simulink model "SimForcesGP2017a"  (R2020b)
settings: Solver=ode4  StartTime=0.0  StopTime=10  FixedStep=0.001  MaxStep=0.001  RelTol=1e-7
values from neighbouring files (symbols this model uses):
  B11_r_B11C = [0.23805608; 0.13201777; 0]    [InitializeSimulationGP.m]
  B11_r_B11Tc1 = [L11; 0; 0]    [InitializeSimulationGP.m]
  B11_Rot_Tc1 = eye(3)    [InitializeSimulationGP.m]
  B11cI = [0.28426000 -0.06487287 0;         -0.06487287  0.54237481 0;                   0  0          0.67891020]    [InitializeSimulationGP.m]
  B12_r_B12C = [0.60504569; 0.27199376; 0.00002484]    [InitializeSimulationGP.m]
  B12_r_B12Tc2 = [L21;0;0]    [InitializeSimulationGP.m]
  B12_Rot_Tc2 = eye(3)    [InitializeSimulationGP.m]
  B12cI = [1.18803886 -2.36786418 0.00280315;          -2.36786418 6.31493281 0.00022322;           0.00280315 0.00022322 7.40915161]    [InitializeSimulationGP.m]
  B31_r_B31C = [0.35781210 0 0]    [InitializeSimulationGP.m]
  B31_Rot_B41 = eye(3)    [InitializeSimulationGP.m]
  B31cI = diag([0.03150902 0.90735702 0.90763033])    [InitializeSimulationGP.m]
  B32_r_B32C = [0.35781210 0 0]    [InitializeSimulationGP.m]
  B32_Rot_B42 = eye(3)    [InitializeSimulationGP.m]
  B32cI = diag([0.03150902 0.90735702 0.90763033])    [InitializeSimulationGP.m]
  B41_r_B41C = [0.55785997 0 0]    [InitializeSimulationGP.m]
  B41_r_B41Tc1 = [lc1;0;0]    [InitializeSimulationGP.m]
  B41cI = diag([0.00370720 0.55759812 0.55785997])    [InitializeSimulationGP.m]
  B42_r_B42C = [0.55785997 0 0]    [InitializeSimulationGP.m]
  B42_r_B42Tc2 = [lc2; 0; 0]    [InitializeSimulationGP.m]
  B42cI = diag([0.00370720 0.55759812 0.55785997])    [InitializeSimulationGP.m]
  B52_r_B52C = [0 0 0.56802906]    [InitializeSimulationGP.m]
  B52_r_B52P32 = [lc3; 0; 0]    [InitializeSimulationGP.m]
  B52_Rot_P32 = eye(3)    [InitializeSimulationGP.m]
  B52cI = diag([0.91789884, 0.91790043, 0.00091463])    [InitializeSimulationGP.m]
  Bc1_r_Bc1B11 = [L1; 0; 0]    [InitializeSimulationGP.m]
  Bc1_r_Bc1B31 = [0;0;0]    [InitializeSimulationGP.m]
  Bc1_r_Bc1C = [0.14178771; 0.16555780; 0]    [InitializeSimulationGP.m]
  Bc1_V = [0;0;0;0;0;0]    [InitializeSimulationGP.m]
  Bc1cI = [+5.892211080 +5.476111360 -0.000019630;          +5.476111360 +28.66965601 -0.000024550;          -0.000019630 -0.000024550 +29.78955950]    [InitializeSimulationGP.m]
  Bc2_r_Bc2B12 = [L2;0;0]    [InitializeSimulationGP.m]
  Bc2_r_Bc2B32 = [0;0;0]    [InitializeSimulationGP.m]
  Bc2_r_Bc2C = [0.54319901; 0.10543875; 0]    [InitializeSimulationGP.m]
  Bc2cI = [0.48071390 0.52924041 0;          0.52924041 5.80912352 0;              0      0          5.97255351]    [InitializeSimulationGP.m]
  beta1 = atan2d(374.261,935)*pi/180    [InitializeSimulationGP.m]
  beta2 = atan2d(45.757,373.313)*pi/180    [InitializeSimulationGP.m]
  beta3 = atan2d(139.50,1132.19)*pi/180    [InitializeSimulationGP.m]
  beta4 = atan2d(88.061,296.198)*pi/180    [InitializeSimulationGP.m]
  D22F = [0;0;0;0;0;0]    [InitializeSimulationGP.m]
  L1 = 1.0071227324212    (= 1.00712273242)    [InitializeSimulationGP.m]
  L11 = 0.37610632101293    (= 0.376106321013)    [InitializeSimulationGP.m]
  L2 = 1.132185817991    (= 1.13218581799)    [InitializeSimulationGP.m]
  L21 = 0.30901132665325    (= 0.309011326653)    [InitializeSimulationGP.m]
  lc1 = 0.745    [InitializeSimulationGP.m]
  lc2 = 0.745    [InitializeSimulationGP.m]
  mB11 = 25.52660174    [InitializeSimulationGP.m]
  mB12 = 33.92850233    [InitializeSimulationGP.m]
  mB31 = 17.36281648    [InitializeSimulationGP.m]
  mB32 = 17.36281648    [InitializeSimulationGP.m]
  mB41 = 10.34519231    [InitializeSimulationGP.m]
  mB42 = 10.34519231    [InitializeSimulationGP.m]
  mB52 = 6.73059863    [InitializeSimulationGP.m]
  mBc1 = 307.29601379    [InitializeSimulationGP.m]
  mBc2 = 54.58702836    [InitializeSimulationGP.m]
  mP22 = 9.26136143    [InitializeSimulationGP.m]
  mP32 = 570.18877059    [InitializeSimulationGP.m]
  P22_r_P22C = [0.62192523 0 0]    [InitializeSimulationGP.m]
  P22_Rot_B52 = eye(3)    [InitializeSimulationGP.m]
  P22cI = diag([0.00662754, 1.48387017, 1.48398069])    [InitializeSimulationGP.m]
  P32_r_P32C = [0.25466704; -0.13034397; -0.01302248]    [InitializeSimulationGP.m]
  P32_r_P32D22 = [0.40499744871392; -0.13130517281345; -0.013385243295654]    [InitializeSimulationGP.m]
  P32_Rot_D22 = [1 0 0;              0 0.9707729441837 0.23999977258512;              0 -0.23999977258512 0.9707729441837]    [InitializeSimulationGP.m]
  P32cI = [46.81220713 0.38607676 -0.00453819;          0.38607676 71.92201786 -1.14320993;          -0.00453819 -1.14320993 67.38128576]    [InitializeSimulationGP.m]
  Tc1_r_Tc1Bc2 = [0.098495302558553; 0.01838181329939; 0]    [InitializeSimulationGP.m]
  Tc1_Rot_Bc2 = [cos(alpha2) -sin(alpha2) 0;                sin(alpha2)  cos(alpha2) 0;                0            0           1]    [InitializeSimulationGP.m]
  Tc2_r_Tc2P22 = [-0.048858374920227;0.36587359346146;0.035276938723102]    [InitializeSimulationGP.m]
  Tc2_Rot_P22 = [0.95853460763586 -0.27664713597974  0.0683942111482;                0.28497614981675  0.93051946315663 -0.23004808784757;                0                 0.23999977258511  0.9707729441837]    [InitializeSimulationGP.m]
  Th1A = 5*pi/180    (= 0.0872664625997)    [InitializeSimulationGP.m]
  Th1B = 20*pi/180    (= 0.349065850399)    [InitializeSimulationGP.m]
  Th1f = 1    [InitializeSimulationGP.m]
  Th2A = 15*pi/180    (= 0.261799387799)    [InitializeSimulationGP.m]
  Th2B = -50*pi/180    (= -0.872664625997)    [InitializeSimulationGP.m]
  Th2f = 2    [InitializeSimulationGP.m]
  W_r_WBc1 = [0.185;-0.085;0]    [InitializeSimulationGP.m]
  W_Rot_Bc1 = [cos(alpha1) -sin(alpha1) 0;              sin(alpha1)  cos(alpha1) 0;              0            0           1]    [InitializeSimulationGP.m]
  Wg = [0; 9.8066; 0]    [InitializeSimulationGP.m]
  x10 = 0.83    [InitializeSimulationGP.m]
  x20 = 0.83    [InitializeSimulationGP.m]
  xf = [1;0;0;0;0;0]    [InitializeSimulationGP.m]
  xt2A = 0.1    [InitializeSimulationGP.m]
  xt2B = 0.5    [InitializeSimulationGP.m]
  xt2f = 1    [InitializeSimulationGP.m]
  ztau = [0;0;0;0;0;1]    [InitializeSimulationGP.m]
undefined symbols (not defined in the file or in its folder): B11_V, B11_V_SS, B11Ftot, B12_U_Tc2, B12_V, B12_V_SS, B12Ftot, B31_r_B31B41, B31_V, B31_V_SS, B31FTot, B32_r_B32B42, B32_U_B42, B32_V, B32_V_SS, B32FTot, B41_V, B41_V_SS, B41FTot, B42_Rot_Tc2, B42_U_Tc2, B42_V, B42_V_SS, B42FTot, B52_U_P32, B52_V, B52_V_SS, B52Ftot, Bc1_V_SS, Bc1Tot, Bc2_Rot_B12, Bc2_Rot_B32, Bc2_U_B12, Bc2_U_B32, Bc2_V, Bc2_V_SS, Bc2Tot, D22_V, D22_V_SS, dq1, dq11, dq12, dq2, dq21, dq22, dx1, dx2, FTot_S1, FTot_S2P, FTot_S2R, P22_r_P22B52, P22_U_B52, P22_V, P22_V_SS, P22FTot, P32_U_D22, P32_V, P32_V_SS, P32FTot, q1 ... (+28)
libraries: nesl_utility x94, sm_lib x45
(part 1 of 5)
settings Model: Creator=liikaneh  LastModifiedBy=Goran
settings OptimizationCC: DefaultParameterBehavior=Inlined  UseFloatMulNetSlope=on  InlineInvariantSignals=on  EfficientFloat2IntCast=on
settings DebuggingCC: ReadBeforeWriteMsg=DisableAll  WriteAfterWriteMsg=DisableAll  WriteAfterReadMsg=DisableAll  MultiTaskDSMMsg=none  ArithmeticOperatorsInVariantConditions=warning
settings ModelReferenceCC: UpdateModelReferenceTargets=IfOutOfDate
settings SFSimCC: SFSimEcho=off  SimUseLocalCustomCode=off  CustomCodeUndefinedFunction=UseInterfaceOnly
settings RTWCC: RTWUseLocalCustomCode=off  BuildConfiguration=Faster Runs
settings CodeAppCC: StateflowObjectComments=on
settings GRTTargetCC: MatFileLogging=off  SupportNonFinite=off
settings DiagnosticsConfigSet: SimMechanicsRigidlyBoundBlock=none

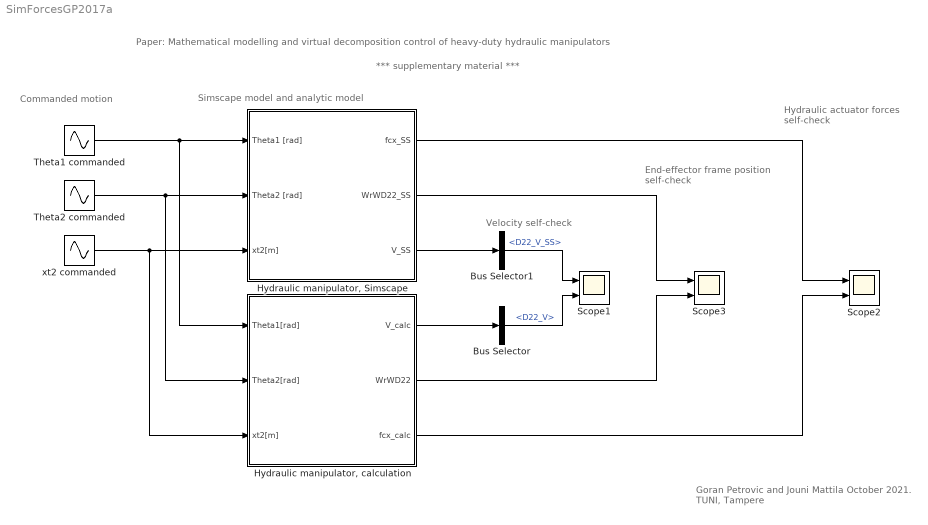
== system SimForcesGP2017a ==
  note: *** supplementary material ***
  note: Paper: Mathematical modelling and virtual decomposition control of heavy-duty hydraulic manipulators
  note: Commanded motion
  note: Simscape model and analytic model
  note: Hydraulic actuator
      | forces self-check
  note: End-effector frame
      | position self-check
  note: Velocity self-check
  note: Goran Petrovic and Jouni Mattila
      | October 2021.
      | TUNI, Tampere
  Bus Selector : BusSelector  OutputSignals=Vels_S2P.D22_V
  Bus Selector1 : BusSelector  OutputSignals=D22_V_SS
  "Hydraulic manipulator, Simscape" : Subsystem
  "Hydraulic manipulator, calculation" : Subsystem
  Scope1 : Scope  NumInputPorts=2
  Scope2 : Scope  NumInputPorts=2
  Scope3 : Scope  NumInputPorts=2
  Theta1 commanded : Sin  Amplitude=Th1A  Bias=Th1B  Frequency=Th1f  SampleTime=0
  Theta2 commanded : Sin  Amplitude=Th2A  Bias=Th2B  Frequency=Th2f  SampleTime=0
  xt2 commanded : Sin  Amplitude=xt2A  Bias=xt2B  Frequency=xt2f  SampleTime=0
  wires:
  xt2 commanded/1 -> "Hydraulic manipulator, calculation"/3(xt2[m]), "Hydraulic manipulator, Simscape"/3(xt2[m])
  Theta1 commanded/1 -> "Hydraulic manipulator, calculation"/1(Theta1[rad]), "Hydraulic manipulator, Simscape"/1(Theta1 [rad])
  Theta2 commanded/1 -> "Hydraulic manipulator, calculation"/2(Theta2[rad]), "Hydraulic manipulator, Simscape"/2(Theta2 [rad])
  "Hydraulic manipulator, calculation"/1(V_calc) -> Bus Selector/1
  "Hydraulic manipulator, Simscape"/3(V_SS) -> Bus Selector1/1
  Bus Selector/1 -> Scope1/2  "<D22_V>"
  Bus Selector1/1 -> Scope1/1  "<D22_V_SS>"
  "Hydraulic manipulator, Simscape"/1(fcx_SS) -> Scope2/1
  "Hydraulic manipulator, calculation"/3(fcx_calc) -> Scope2/2
  "Hydraulic manipulator, Simscape"/2(WrWD22_SS) -> Scope3/1
  "Hydraulic manipulator, calculation"/2(WrWD22) -> Scope3/2

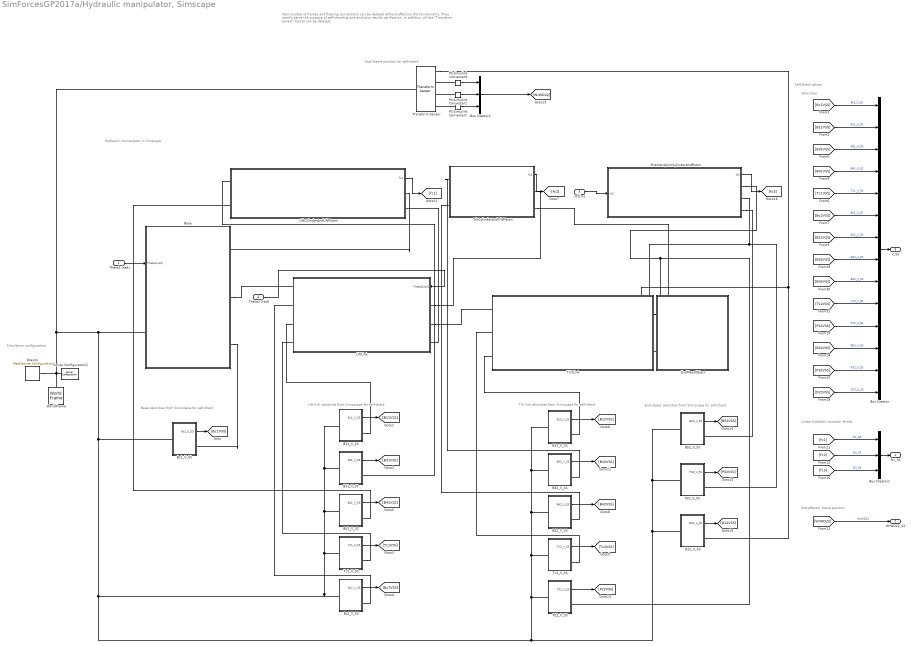
== system SimForcesGP2017a/Hydraulic manipulator, Simscape ==
  note: Vast number of frames and floating connections can be deleted without affecting the functionality.
      | They mainly serve the purpose of self-checking and analytics results verification.
      | In addition, all the "Transform sensor" blocks can be deleted.
  note: Hydraulic manipulator in Simscape
  note: Simulation configuration
  note: End object velocities from Simcscape for self-check
  note: Tilt link velocities from Simcscape for self-check
  note: Base velocities from Simcscape for self-check
  note: Lift link velocities from Simcscape for self-check
  note: Self-check values
  note: Velocities
  note: Linear hydraulic actuator forces
  note: End-effector frame position
  note: Goal frame position for self-check
  Theta1 [rad] : Inport
  Theta2 [rad] : Inport  Port=2
  xt2[m] : Inport  Port=3
  B11_V_SS : Subsystem
  B12_V_SS : Subsystem
  B31_V_SS : Subsystem
  B32_V_SS : Subsystem
  B41_V_SS : Subsystem
  B42_V_SS : Subsystem
  B52_V_SS : Subsystem
  Base : Subsystem
  Bc1_V_SS : Subsystem
  Bc2_V_SS : Subsystem
  Bus Creator : BusCreator  Inputs=Bc1_V_SS,B11_V_SS,B31_V_SS,B41_V_SS,Tc1_V_SS,Bc2_V_SS,B12_V_SS,B32_V_SS,B42_V_SS,Tc2_V_SS,P22_V_SS,B52_V_SS,P32_V_SS,D22_V_SS
  Bus Creator1 : BusCreator  Inputs=3
  Bus Creator2 : BusCreator  Inputs=3
  D22_V_SS : Subsystem
  EndMassObject : Subsystem
  Gravity : sm_lib/Utilities/Mechanism Configuration  UniformGravity=Constant  GravityVector=-Wg  GravityVectorUnits=m/s^2  GravityUnits=m/s^2  LinearizationDelta=0.001  JointModeTransitionNonlinearIterations=2
  LiftCylinderAndLiftPiston : Subsystem
  LiftLink : Subsystem
  P22_V_SS : Subsystem
  P32_V_SS : Subsystem
  PS-Simulink Converter1 : nesl_utility/PS-Simulink Converter  PhysicalDomain=network_engine_domain  SubClassName=ps_output  LeftPortType=input  RightPortType=output  PseudoPeriodic=off  Frequencies=[]  Unit=inherit  AffineConversion=off
  PS-Simulink Converter2 : nesl_utility/PS-Simulink Converter  PhysicalDomain=network_engine_domain  SubClassName=ps_output  LeftPortType=input  RightPortType=output  PseudoPeriodic=off  Frequencies=[]  Unit=inherit  AffineConversion=off
  PS-Simulink Converter8 : nesl_utility/PS-Simulink Converter  PhysicalDomain=network_engine_domain  SubClassName=ps_output  LeftPortType=input  RightPortType=output  PseudoPeriodic=off  Frequencies=[]  Unit=inherit  AffineConversion=off
  PrismaticJointCylinderAndPiston : Subsystem
  Solver Configuration1 : nesl_utility/Solver Configuration  PhysicalDomain=network_engine_domain  SubClassName=solver  LeftPortType=input  RightPortType=generic  Tones=[]  Harmonics=[]  SimulateNoise=off  Profile=off  UseLocalSampling=off  EnableSwitchedLinearOptims=on  FrequencyDomain=off  UseCCode=off  RelTol=0.001  AbsTol=1e-06  MinStep=1e-09  ToWorkspace=off  RevertToSquareIcSolve=off  NumHomotopyIterations=100  PhasorMode=off  PhasorModeNumHarmonics=1  DoDC=on  ResidualTolerance=1e-9  UseLocalSolver=off  LocalSolverChoice=NE_TRAPEZOIDAL_ADVANCER  LocalSolverSampleTime=0.002  DoFixedCost=off  MaxNonlinIter=3  MaxModeIter=2  ComputeImpulses=off  ImpulseIterations=2  LinearAlgebra=Sparse  EquationFormulation=NE_TIME_EF  DelaysMemoryBudget=1024  AutomaticFiltering=on  FilteringTimeConstant=0.001  PartitionStorageMethod=AS_NEEDED  PartitionMemoryBudget=1024  PartitionMethod=FAST
  Tc1_V_SS : Subsystem
  Tc2_V_SS : Subsystem
  TilitLink : Subsystem
  TiltCylinderAndTiltPiston : Subsystem
  Transform Sensor : sm_lib/Frames and Transforms/Transform Sensor  MeasurementFrame=NonRotatingBase  SenseAngle=off  SenseAxis=off  SenseAngle1=off  SenseAngle2=off  SenseAngle3=off  SenseQ=off  SenseR=off  SenseOmegaX=off  SenseOmegaY=off  SenseOmegaZ=off  SenseOmega1=off  SenseOmega2=off  SenseOmega3=off  SenseQDot=off  SenseRDot=off  SenseAlphaX=off  SenseAlphaY=off  SenseAlphaZ=off  SenseAlpha1=off  SenseAlpha2=off  SenseAlpha3=off  SenseQDDot=off  SenseRDDot=off  SenseX=on  SenseY=on  SenseZ=on  SenseRad=off  SenseAzim=off  SenseDist=off  SenseInc=off  SenseXDot=off  SenseYDot=off  SenseZDot=off  SenseRadDot=off  SenseAzimDot=off  SenseDistDot=off  SenseIncDot=off  SenseXDDot=off  SenseYDDot=off  SenseZDDot=off  SenseRadDDot=off  SenseAzimDDot=off  SenseDistDDot=off  SenseIncDDot=off
  WorldFrame : sm_lib/Frames and Transforms/World Frame
  fcx_SS : Outport
  WrWD22_SS : Outport  Port=2
  V_SS : Outport  Port=3
  wires:
  LiftCylinderAndLiftPiston/1(fc1) -> [fc1]
  TiltCylinderAndTiltPiston/1(fc2) -> [fc2]
  xt2[m]/1 -> PrismaticJointCylinderAndPiston/1(xt2)
  PrismaticJointCylinderAndPiston/1(fc3) -> [fc3]
  Theta1 [rad]/1 -> Base/1(Theta1[rad])
  Theta2 [rad]/1 -> LiftLink/1(Theta2[rad])
  B11_V_SS/1(B11_V_SS) -> [B11VSS]
  B41_V_SS/1(B41_V_SS) -> [B41VSS]
  B52_V_SS/1(B52_V_SS) -> [B52VSS]
  Bc1_V_SS/1(Bc1_V_SS) -> [Bc1VSS]
  B12_V_SS/1(B12_V_SS) -> [B12VSS]
  P32_V_SS/1(P32_V_SS) -> [P32VSS]
  P22_V_SS/1(P22_V_SS) -> [P22VSS]
  Tc2_V_SS/1(Tc2_V_SS) -> [Tc2VSS]
  B31_V_SS/1(B31_V_SS) -> [B31VSS]
  B42_V_SS/1(B42_V_SS) -> [B42VSS]
  D22_V_SS/1(D22_V_SS) -> [D22VSS]
  Bc2_V_SS/1(Bc2_V_SS) -> [Bc2VSS]
  Tc1_V_SS/1(Tc1_V_SS) -> [Tc1VSS]
  B32_V_SS/1(B32_V_SS) -> [B32VSS]
  [B12VSS] -> Bus Creator/7  "B12_V_SS"
  [B42VSS] -> Bus Creator/9  "B42_V_SS"
  [Tc2VSS] -> Bus Creator/10  "Tc2_V_SS"
  [fc1] -> Bus Creator1/1  "fc1_SS"
  Bus Creator/1 -> V_SS/1
  [P32VSS] -> Bus Creator/13  "P32_V_SS"
  [B32VSS] -> Bus Creator/8  "B32_V_SS"
  [fc2] -> Bus Creator1/2  "fc2_SS"
  [fc3] -> Bus Creator1/3  "fc3_SS"
  [WrWD22] -> WrWD22_SS/1  "WrWD22"
  Bus Creator1/1 -> fcx_SS/1
  [B52VSS] -> Bus Creator/12  "B52_V_SS"
  [P22VSS] -> Bus Creator/11  "P22_V_SS"
  [D22VSS] -> Bus Creator/14  "D22_V_SS"
  [Bc1VSS] -> Bus Creator/1  "Bc1_V_SS"
  [B11VSS] -> Bus Creator/2  "B11_V_SS"
  [Tc1VSS] -> Bus Creator/5  "Tc1_V_SS"
  [B41VSS] -> Bus Creator/4  "B41_V_SS"
  [B31VSS] -> Bus Creator/3  "B31_V_SS"
  [Bc2VSS] -> Bus Creator/6  "Bc2_V_SS"
  PS-Simulink Converter2/1 -> Bus Creator2/3
  PS-Simulink Converter8/1 -> Bus Creator2/1
  PS-Simulink Converter1/1 -> Bus Creator2/2
  Bus Creator2/1 -> [WrWD22]
  connections:
  P32_V_SS/LConn1 -- B52_V_SS/LConn1 -- Gravity/RConn1 -- WorldFrame/RConn1 -- Solver Configuration1/RConn1 -- Transform Sensor/LConn1 -- Base/LConn1 -- Bc1_V_SS/LConn1 -- B41_V_SS/LConn1 -- B31_V_SS/LConn1 -- B11_V_SS/LConn1 -- Tc1_V_SS/LConn1 -- Bc2_V_SS/LConn1 -- B32_V_SS/LConn1 -- B12_V_SS/LConn1 -- B42_V_SS/LConn1 -- Tc2_V_SS/LConn1 -- P22_V_SS/LConn1 -- D22_V_SS/LConn1
  LiftLink/LConn1 -- TiltCylinderAndTiltPiston/RConn1
  LiftLink/LConn2 -- TilitLink/RConn1
  TiltCylinderAndTiltPiston/RConn2 -- TilitLink/LConn2
  LiftCylinderAndLiftPiston/RConn2 -- LiftLink/LConn3
  Base/RConn2 -- LiftLink/RConn1
  LiftCylinderAndLiftPiston/RConn1 -- Base/RConn1
  Tc1_V_SS/RConn1 -- LiftLink/RConn4
  PrismaticJointCylinderAndPiston/RConn2 -- EndMassObject/LConn1 -- P32_V_SS/RConn1
  EndMassObject/LConn2 -- Transform Sensor/RConn1 -- D22_V_SS/RConn1
  LiftCylinderAndLiftPiston/LConn2 -- B41_V_SS/RConn1
  B11_V_SS/RConn1 -- LiftLink/RConn3
  TiltCylinderAndTiltPiston/LConn2 -- B42_V_SS/RConn1
  TiltCylinderAndTiltPiston/LConn1 -- B32_V_SS/RConn1
  PrismaticJointCylinderAndPiston/RConn1 -- P22_V_SS/RConn1 -- TilitLink/LConn1
  LiftCylinderAndLiftPiston/LConn1 -- B31_V_SS/RConn1
  TilitLink/RConn3 -- B12_V_SS/RConn1
  PrismaticJointCylinderAndPiston/RConn3 -- B52_V_SS/RConn1
  LiftLink/RConn2 -- Bc2_V_SS/RConn1
  Tc2_V_SS/RConn1 -- TilitLink/RConn2
  Base/RConn3 -- Bc1_V_SS/RConn1
  PS-Simulink Converter1/LConn1 -- Transform Sensor/RConn3
  PS-Simulink Converter8/LConn1 -- Transform Sensor/RConn2
  PS-Simulink Converter2/LConn1 -- Transform Sensor/RConn4

== system SimForcesGP2017a/Hydraulic manipulator, calculation ==
  note: Pass to outputs...
  note: Get inputs...
  note: Process data...
  Theta1[rad] : Inport
  Theta2[rad] : Inport  Port=2
  xt2[m] : Inport  Port=3
  AnalyticEnd-EffectorFramePosition : Subsystem
  AnalyticForces : Subsystem
  AnalyticTotalForces : Subsystem
  AnalyticVelocities : Subsystem
  AngleRelations : Subsystem
  Constant1 : Constant  Value=Bc1_V
  D22F : Constant  Value=D22F
  V_calc : Outport
  WrWD22 : Outport  Port=2
  fcx_calc : Outport  Port=3
  wires:
  AnalyticTotalForces/1(FTot_Sx) -> [FTot_Sx]
  AnalyticVelocities/1(GeomProp_Sx) -> [GeomSx]
  AnalyticVelocities/4(UMat_Sx) -> [UMatsSx]
  [UMatsSx] -> AnalyticForces/2(UMatSx)
  [VelsSx] -> AnalyticTotalForces/1(Vels_Sx)
  [GeomSx] -> AnalyticForces/3(GeomCCx)
  AnalyticVelocities/3(WRotX_Sx) -> [WRotXSx]
  [WRotXSx] -> AnalyticTotalForces/2(WRotX_Sx)
  [FTot_Sx] -> AnalyticForces/1(Ftot_Sx)
  AnalyticVelocities/5(Vels_Sx) -> [VelsSx]
  Theta1[rad]/1 -> [Theta1]  "Theta1"
  Theta2[rad]/1 -> [Theta2]  "Theta2"
  [Theta1] -> AngleRelations/1(Theta1[rad])  "Theta1"
  [Theta2] -> AngleRelations/2(Theta2[rad])  "Theta2"
  AngleRelations/1(q1[rad]) -> [q1]  "q1"
  AngleRelations/2(q2[rad]) -> [q2]  "q2"
  [q2] -> AnalyticVelocities/2(q2[rad])  "q2"
  [q1] -> AnalyticVelocities/1(q1[rad])  "q1"
  AnalyticForces/1(fc) -> [fc]
  [fc] -> fcx_calc/1
  [VelsSx] -> V_calc/1
  [D22F] -> AnalyticForces/4(GF)
  [WRotXSx] -> AnalyticEnd-EffectorFramePosition/2(WRotX_Sx)
  AnalyticVelocities/2(PosVecs_Sx) -> [PosVecsSx]
  [PosVecsSx] -> AnalyticEnd-EffectorFramePosition/1(PosVecs_Sx)
  AnalyticEnd-EffectorFramePosition/1(WrWD22) -> [WrWD22]
  [WrWD22] -> WrWD22/1
  D22F/1 -> [D22F]  "D22F"
  xt2[m]/1 -> [xt2]  "xt2"
  [xt2] -> AnalyticVelocities/3(xt2[m])  "x3"
  Constant1/1 -> [Bc1V]  "Bc1_V"
  [Bc1V] -> AnalyticVelocities/4(Bc1V)

== system SimForcesGP2017a/Hydraulic manipulator, Simscape/B11_V_SS ==
  Mux3 : Mux  Inputs=6
  PS-Simulink Converter{1..3,7..9} (6 alike) : nesl_utility/PS-Simulink Converter  PhysicalDomain=network_engine_domain  SubClassName=ps_output  LeftPortType=input  RightPortType=output  PseudoPeriodic=off  Frequencies=[]  Unit=inherit  AffineConversion=off
  Selector : Selector  InputPortWidth=6  IndexOptions=Index vector (dialog)  Indices=[4 5 6 1 2 3]  OutputSizes=1
  Transform Sensor3 : sm_lib/Frames and Transforms/Transform Sensor  MeasurementFrame=NonRotatingFollower  SenseAngle=off  SenseAxis=off  SenseAngle1=off  SenseAngle2=off  SenseAngle3=off  SenseQ=off  SenseR=off  SenseOmegaX=on  SenseOmegaY=on  SenseOmegaZ=on  SenseOmega1=off  SenseOmega2=off  SenseOmega3=off  SenseQDot=off  SenseRDot=off  SenseAlphaX=off  SenseAlphaY=off  SenseAlphaZ=off  SenseAlpha1=off  SenseAlpha2=off  SenseAlpha3=off  SenseQDDot=off  SenseRDDot=off  SenseX=off  SenseY=off  SenseZ=off  SenseRad=off  SenseAzim=off  SenseDist=off  SenseInc=off  SenseXDot=on  SenseYDot=on  SenseZDot=on  SenseRadDot=off  SenseAzimDot=off  SenseDistDot=off  SenseIncDot=off  SenseXDDot=off  SenseYDDot=off  SenseZDDot=off  SenseRadDDot=off  SenseAzimDDot=off  SenseDistDDot=off  SenseIncDDot=off
  Lift_B11 : PMIOPort  Side=Right
  W : PMIOPort  Port=2  Side=Left
  B11_V_SS : Outport
  wires:
  Mux3/1 -> Selector/1
  PS-Simulink Converter7/1 -> Mux3/2
  PS-Simulink Converter3/1 -> Mux3/6
  PS-Simulink Converter2/1 -> Mux3/5
  PS-Simulink Converter9/1 -> Mux3/1
  PS-Simulink Converter8/1 -> Mux3/3
  PS-Simulink Converter1/1 -> Mux3/4
  Selector/1 -> B11_V_SS/1
  connections:
  Transform Sensor3/RConn5 -- PS-Simulink Converter1/LConn1
  PS-Simulink Converter3/LConn1 -- Transform Sensor3/RConn7
  Transform Sensor3/LConn1 -- W/RConn1
  Transform Sensor3/RConn4 -- PS-Simulink Converter8/LConn1
  PS-Simulink Converter7/LConn1 -- Transform Sensor3/RConn3
  PS-Simulink Converter9/LConn1 -- Transform Sensor3/RConn2
  Transform Sensor3/RConn6 -- PS-Simulink Converter2/LConn1
  Transform Sensor3/RConn1 -- Lift_B11/RConn1

== system SimForcesGP2017a/Hydraulic manipulator, Simscape/B12_V_SS ==
  Mux3 : Mux  Inputs=6
  PS-Simulink Converter{1..3,7..9} (6 alike) : nesl_utility/PS-Simulink Converter  PhysicalDomain=network_engine_domain  SubClassName=ps_output  LeftPortType=input  RightPortType=output  PseudoPeriodic=off  Frequencies=[]  Unit=inherit  AffineConversion=off
  Selector1 : Selector  InputPortWidth=6  IndexOptions=Index vector (dialog)  Indices=[4 5 6 1 2 3]  OutputSizes=1
  Transform Sensor1 : sm_lib/Frames and Transforms/Transform Sensor  MeasurementFrame=NonRotatingFollower  SenseAngle=off  SenseAxis=off  SenseAngle1=off  SenseAngle2=off  SenseAngle3=off  SenseQ=off  SenseR=off  SenseOmegaX=on  SenseOmegaY=on  SenseOmegaZ=on  SenseOmega1=off  SenseOmega2=off  SenseOmega3=off  SenseQDot=off  SenseRDot=off  SenseAlphaX=off  SenseAlphaY=off  SenseAlphaZ=off  SenseAlpha1=off  SenseAlpha2=off  SenseAlpha3=off  SenseQDDot=off  SenseRDDot=off  SenseX=off  SenseY=off  SenseZ=off  SenseRad=off  SenseAzim=off  SenseDist=off  SenseInc=off  SenseXDot=on  SenseYDot=on  SenseZDot=on  SenseRadDot=off  SenseAzimDot=off  SenseDistDot=off  SenseIncDot=off  SenseXDDot=off  SenseYDDot=off  SenseZDDot=off  SenseRadDDot=off  SenseAzimDDot=off  SenseDistDDot=off  SenseIncDDot=off
  Tilt_B12 : PMIOPort  Side=Right
  W : PMIOPort  Port=2  Side=Left
  B12_V_SS : Outport
  wires:
  PS-Simulink Converter1/1 -> Mux3/4
  PS-Simulink Converter8/1 -> Mux3/3
  PS-Simulink Converter9/1 -> Mux3/1
  PS-Simulink Converter2/1 -> Mux3/5
  PS-Simulink Converter3/1 -> Mux3/6
  PS-Simulink Converter7/1 -> Mux3/2
  Mux3/1 -> Selector1/1
  Selector1/1 -> B12_V_SS/1
  connections:
  Transform Sensor1/RConn1 -- Tilt_B12/RConn1
  Transform Sensor1/RConn6 -- PS-Simulink Converter2/LConn1
  Transform Sensor1/RConn2 -- PS-Simulink Converter9/LConn1
  Transform Sensor1/RConn3 -- PS-Simulink Converter7/LConn1
  Transform Sensor1/RConn4 -- PS-Simulink Converter8/LConn1
  Transform Sensor1/LConn1 -- W/RConn1
  Transform Sensor1/RConn7 -- PS-Simulink Converter3/LConn1
  Transform Sensor1/RConn5 -- PS-Simulink Converter1/LConn1

== system SimForcesGP2017a/Hydraulic manipulator, Simscape/B31_V_SS ==
  Mux3 : Mux  Inputs=6
  PS-Simulink Converter{1..3,7..9} (6 alike) : nesl_utility/PS-Simulink Converter  PhysicalDomain=network_engine_domain  SubClassName=ps_output  LeftPortType=input  RightPortType=output  PseudoPeriodic=off  Frequencies=[]  Unit=inherit  AffineConversion=off
  Selector1 : Selector  InputPortWidth=6  IndexOptions=Index vector (dialog)  Indices=[4 5 6 1 2 3]  OutputSizes=1
  Transform Sensor1 : sm_lib/Frames and Transforms/Transform Sensor  MeasurementFrame=NonRotatingFollower  SenseAngle=off  SenseAxis=off  SenseAngle1=off  SenseAngle2=off  SenseAngle3=off  SenseQ=off  SenseR=off  SenseOmegaX=on  SenseOmegaY=on  SenseOmegaZ=on  SenseOmega1=off  SenseOmega2=off  SenseOmega3=off  SenseQDot=off  SenseRDot=off  SenseAlphaX=off  SenseAlphaY=off  SenseAlphaZ=off  SenseAlpha1=off  SenseAlpha2=off  SenseAlpha3=off  SenseQDDot=off  SenseRDDot=off  SenseX=off  SenseY=off  SenseZ=off  SenseRad=off  SenseAzim=off  SenseDist=off  SenseInc=off  SenseXDot=on  SenseYDot=on  SenseZDot=on  SenseRadDot=off  SenseAzimDot=off  SenseDistDot=off  SenseIncDot=off  SenseXDDot=off  SenseYDDot=off  SenseZDDot=off  SenseRadDDot=off  SenseAzimDDot=off  SenseDistDDot=off  SenseIncDDot=off
  Lift_B31 : PMIOPort  Side=Right
  W : PMIOPort  Port=2  Side=Left
  B31_V_SS : Outport
  wires:
  Mux3/1 -> Selector1/1
  PS-Simulink Converter7/1 -> Mux3/2
  PS-Simulink Converter3/1 -> Mux3/6
  PS-Simulink Converter2/1 -> Mux3/5
  PS-Simulink Converter9/1 -> Mux3/1
  PS-Simulink Converter8/1 -> Mux3/3
  PS-Simulink Converter1/1 -> Mux3/4
  Selector1/1 -> B31_V_SS/1
  connections:
  Transform Sensor1/RConn5 -- PS-Simulink Converter1/LConn1
  Transform Sensor1/RConn7 -- PS-Simulink Converter3/LConn1
  Transform Sensor1/LConn1 -- W/RConn1
  Transform Sensor1/RConn4 -- PS-Simulink Converter8/LConn1
  Transform Sensor1/RConn3 -- PS-Simulink Converter7/LConn1
  Transform Sensor1/RConn2 -- PS-Simulink Converter9/LConn1
  Transform Sensor1/RConn6 -- PS-Simulink Converter2/LConn1
  Transform Sensor1/RConn1 -- Lift_B31/RConn1

== system SimForcesGP2017a/Hydraulic manipulator, Simscape/B32_V_SS ==
  Mux3 : Mux  Inputs=6
  PS-Simulink Converter{1..3,7..9} (6 alike) : nesl_utility/PS-Simulink Converter  PhysicalDomain=network_engine_domain  SubClassName=ps_output  LeftPortType=input  RightPortType=output  PseudoPeriodic=off  Frequencies=[]  Unit=inherit  AffineConversion=off
  Selector1 : Selector  InputPortWidth=6  IndexOptions=Index vector (dialog)  Indices=[4 5 6 1 2 3]  OutputSizes=1
  Transform Sensor1 : sm_lib/Frames and Transforms/Transform Sensor  MeasurementFrame=NonRotatingFollower  SenseAngle=off  SenseAxis=off  SenseAngle1=off  SenseAngle2=off  SenseAngle3=off  SenseQ=off  SenseR=off  SenseOmegaX=on  SenseOmegaY=on  SenseOmegaZ=on  SenseOmega1=off  SenseOmega2=off  SenseOmega3=off  SenseQDot=off  SenseRDot=off  SenseAlphaX=off  SenseAlphaY=off  SenseAlphaZ=off  SenseAlpha1=off  SenseAlpha2=off  SenseAlpha3=off  SenseQDDot=off  SenseRDDot=off  SenseX=off  SenseY=off  SenseZ=off  SenseRad=off  SenseAzim=off  SenseDist=off  SenseInc=off  SenseXDot=on  SenseYDot=on  SenseZDot=on  SenseRadDot=off  SenseAzimDot=off  SenseDistDot=off  SenseIncDot=off  SenseXDDot=off  SenseYDDot=off  SenseZDDot=off  SenseRadDDot=off  SenseAzimDDot=off  SenseDistDDot=off  SenseIncDDot=off
  Tilt_B32 : PMIOPort  Side=Right
  W : PMIOPort  Port=2  Side=Left
  B32_V_SS : Outport
  wires:
  Mux3/1 -> Selector1/1
  PS-Simulink Converter7/1 -> Mux3/2
  PS-Simulink Converter3/1 -> Mux3/6
  PS-Simulink Converter2/1 -> Mux3/5
  PS-Simulink Converter9/1 -> Mux3/1
  PS-Simulink Converter8/1 -> Mux3/3
  PS-Simulink Converter1/1 -> Mux3/4
  Selector1/1 -> B32_V_SS/1
  connections:
  Transform Sensor1/RConn5 -- PS-Simulink Converter1/LConn1
  Transform Sensor1/RConn7 -- PS-Simulink Converter3/LConn1
  Transform Sensor1/LConn1 -- W/RConn1
  Transform Sensor1/RConn4 -- PS-Simulink Converter8/LConn1
  Transform Sensor1/RConn3 -- PS-Simulink Converter7/LConn1
  Transform Sensor1/RConn2 -- PS-Simulink Converter9/LConn1
  Transform Sensor1/RConn6 -- PS-Simulink Converter2/LConn1
  Transform Sensor1/RConn1 -- Tilt_B32/RConn1

== system SimForcesGP2017a/Hydraulic manipulator, Simscape/B41_V_SS ==
  Mux3 : Mux  Inputs=6
  PS-Simulink Converter{1..3,7..9} (6 alike) : nesl_utility/PS-Simulink Converter  PhysicalDomain=network_engine_domain  SubClassName=ps_output  LeftPortType=input  RightPortType=output  PseudoPeriodic=off  Frequencies=[]  Unit=inherit  AffineConversion=off
  Selector1 : Selector  InputPortWidth=6  IndexOptions=Index vector (dialog)  Indices=[4 5 6 1 2 3]  OutputSizes=1
  Transform Sensor1 : sm_lib/Frames and Transforms/Transform Sensor  MeasurementFrame=NonRotatingFollower  SenseAngle=off  SenseAxis=off  SenseAngle1=off  SenseAngle2=off  SenseAngle3=off  SenseQ=off  SenseR=off  SenseOmegaX=on  SenseOmegaY=on  SenseOmegaZ=on  SenseOmega1=off  SenseOmega2=off  SenseOmega3=off  SenseQDot=off  SenseRDot=off  SenseAlphaX=off  SenseAlphaY=off  SenseAlphaZ=off  SenseAlpha1=off  SenseAlpha2=off  SenseAlpha3=off  SenseQDDot=off  SenseRDDot=off  SenseX=off  SenseY=off  SenseZ=off  SenseRad=off  SenseAzim=off  SenseDist=off  SenseInc=off  SenseXDot=on  SenseYDot=on  SenseZDot=on  SenseRadDot=off  SenseAzimDot=off  SenseDistDot=off  SenseIncDot=off  SenseXDDot=off  SenseYDDot=off  SenseZDDot=off  SenseRadDDot=off  SenseAzimDDot=off  SenseDistDDot=off  SenseIncDDot=off
  Lift_B41 : PMIOPort  Side=Right
  W : PMIOPort  Port=2  Side=Left
  B41_V_SS : Outport
  wires:
  PS-Simulink Converter1/1 -> Mux3/4
  PS-Simulink Converter8/1 -> Mux3/3
  PS-Simulink Converter9/1 -> Mux3/1
  PS-Simulink Converter2/1 -> Mux3/5
  PS-Simulink Converter3/1 -> Mux3/6
  PS-Simulink Converter7/1 -> Mux3/2
  Mux3/1 -> Selector1/1
  Selector1/1 -> B41_V_SS/1
  connections:
  Transform Sensor1/RConn1 -- Lift_B41/RConn1
  Transform Sensor1/RConn6 -- PS-Simulink Converter2/LConn1
  Transform Sensor1/RConn2 -- PS-Simulink Converter9/LConn1
  Transform Sensor1/RConn3 -- PS-Simulink Converter7/LConn1
  Transform Sensor1/RConn4 -- PS-Simulink Converter8/LConn1
  Transform Sensor1/LConn1 -- W/RConn1
  Transform Sensor1/RConn7 -- PS-Simulink Converter3/LConn1
  Transform Sensor1/RConn5 -- PS-Simulink Converter1/LConn1

== system SimForcesGP2017a/Hydraulic manipulator, Simscape/B42_V_SS ==
  Mux3 : Mux  Inputs=6
  PS-Simulink Converter{1..3,7..9} (6 alike) : nesl_utility/PS-Simulink Converter  PhysicalDomain=network_engine_domain  SubClassName=ps_output  LeftPortType=input  RightPortType=output  PseudoPeriodic=off  Frequencies=[]  Unit=inherit  AffineConversion=off
  Selector1 : Selector  InputPortWidth=6  IndexOptions=Index vector (dialog)  Indices=[4 5 6 1 2 3]  OutputSizes=1
  Transform Sensor1 : sm_lib/Frames and Transforms/Transform Sensor  MeasurementFrame=NonRotatingFollower  SenseAngle=off  SenseAxis=off  SenseAngle1=off  SenseAngle2=off  SenseAngle3=off  SenseQ=off  SenseR=off  SenseOmegaX=on  SenseOmegaY=on  SenseOmegaZ=on  SenseOmega1=off  SenseOmega2=off  SenseOmega3=off  SenseQDot=off  SenseRDot=off  SenseAlphaX=off  SenseAlphaY=off  SenseAlphaZ=off  SenseAlpha1=off  SenseAlpha2=off  SenseAlpha3=off  SenseQDDot=off  SenseRDDot=off  SenseX=off  SenseY=off  SenseZ=off  SenseRad=off  SenseAzim=off  SenseDist=off  SenseInc=off  SenseXDot=on  SenseYDot=on  SenseZDot=on  SenseRadDot=off  SenseAzimDot=off  SenseDistDot=off  SenseIncDot=off  SenseXDDot=off  SenseYDDot=off  SenseZDDot=off  SenseRadDDot=off  SenseAzimDDot=off  SenseDistDDot=off  SenseIncDDot=off
  Tilt_B42 : PMIOPort  Side=Right
  W : PMIOPort  Port=2  Side=Left
  B42_V_SS : Outport
  wires:
  PS-Simulink Converter1/1 -> Mux3/4
  PS-Simulink Converter8/1 -> Mux3/3
  PS-Simulink Converter9/1 -> Mux3/1
  PS-Simulink Converter2/1 -> Mux3/5
  PS-Simulink Converter3/1 -> Mux3/6
  PS-Simulink Converter7/1 -> Mux3/2
  Mux3/1 -> Selector1/1
  Selector1/1 -> B42_V_SS/1
  connections:
  Transform Sensor1/RConn1 -- Tilt_B42/RConn1
  Transform Sensor1/RConn6 -- PS-Simulink Converter2/LConn1
  Transform Sensor1/RConn2 -- PS-Simulink Converter9/LConn1
  Transform Sensor1/RConn3 -- PS-Simulink Converter7/LConn1
  Transform Sensor1/RConn4 -- PS-Simulink Converter8/LConn1
  Transform Sensor1/LConn1 -- W/RConn1
  Transform Sensor1/RConn7 -- PS-Simulink Converter3/LConn1
  Transform Sensor1/RConn5 -- PS-Simulink Converter1/LConn1

== system SimForcesGP2017a/Hydraulic manipulator, Simscape/B52_V_SS ==
  Mux3 : Mux  Inputs=6
  PS-Simulink Converter{1..3,7..9} (6 alike) : nesl_utility/PS-Simulink Converter  PhysicalDomain=network_engine_domain  SubClassName=ps_output  LeftPortType=input  RightPortType=output  PseudoPeriodic=off  Frequencies=[]  Unit=inherit  AffineConversion=off
  Selector1 : Selector  InputPortWidth=6  IndexOptions=Index vector (dialog)  Indices=[4 5 6 1 2 3]  OutputSizes=1
  Transform Sensor1 : sm_lib/Frames and Transforms/Transform Sensor  MeasurementFrame=NonRotatingFollower  SenseAngle=off  SenseAxis=off  SenseAngle1=off  SenseAngle2=off  SenseAngle3=off  SenseQ=off  SenseR=off  SenseOmegaX=on  SenseOmegaY=on  SenseOmegaZ=on  SenseOmega1=off  SenseOmega2=off  SenseOmega3=off  SenseQDot=off  SenseRDot=off  SenseAlphaX=off  SenseAlphaY=off  SenseAlphaZ=off  SenseAlpha1=off  SenseAlpha2=off  SenseAlpha3=off  SenseQDDot=off  SenseRDDot=off  SenseX=off  SenseY=off  SenseZ=off  SenseRad=off  SenseAzim=off  SenseDist=off  SenseInc=off  SenseXDot=on  SenseYDot=on  SenseZDot=on  SenseRadDot=off  SenseAzimDot=off  SenseDistDot=off  SenseIncDot=off  SenseXDDot=off  SenseYDDot=off  SenseZDDot=off  SenseRadDDot=off  SenseAzimDDot=off  SenseDistDDot=off  SenseIncDDot=off
  Obj_B52 : PMIOPort  Side=Right
  W : PMIOPort  Port=2  Side=Left
  B52_V_SS : Outport
  wires:
  Selector1/1 -> B52_V_SS/1
  Mux3/1 -> Selector1/1
  PS-Simulink Converter7/1 -> Mux3/2
  PS-Simulink Converter3/1 -> Mux3/6
  PS-Simulink Converter2/1 -> Mux3/5
  PS-Simulink Converter9/1 -> Mux3/1
  PS-Simulink Converter8/1 -> Mux3/3
  PS-Simulink Converter1/1 -> Mux3/4
  connections:
  Transform Sensor1/RConn5 -- PS-Simulink Converter1/LConn1
  Transform Sensor1/RConn7 -- PS-Simulink Converter3/LConn1
  Transform Sensor1/LConn1 -- W/RConn1
  Transform Sensor1/RConn4 -- PS-Simulink Converter8/LConn1
  Transform Sensor1/RConn3 -- PS-Simulink Converter7/LConn1
  Transform Sensor1/RConn2 -- PS-Simulink Converter9/LConn1
  Transform Sensor1/RConn6 -- PS-Simulink Converter2/LConn1
  Transform Sensor1/RConn1 -- Obj_B52/RConn1

== system SimForcesGP2017a/Hydraulic manipulator, Simscape/Base ==
  note: Analytic derivatives
  note: Define world (W) frame.
  Theta1[rad] : Inport
  BaseR_To_W : sm_lib/Frames and Transforms/Rigid Transform  TranslationMethod=None  TranslationStandardOffset=0  TranslationLengthUnit=m  TranslationStandardAxis=+Z  TranslationCartesianOffset=[0 0 0]  TranslationROffset=0  TranslationROffsetUnits=m  TranslationZOffset=0  TranslationZOffsetUnits=m  TranslationThetaOffset=0  TranslationThetaOffsetUnits=deg  RotationMethod=StandardAxis  RotationAngleUnits=deg  RotationStandardAxis=+Y  RotationAngle=90  RotationArbitraryAxis=[0 0 1]  FollAlignAxisA=+X  BaseAlignAxisA=+Y  FollAlignAxisB=+Y  BaseAlignAxisB=+Z  RotationSequenceAxes=FollowerAxes  RotationSequence=XYX  RotationSequenceAngles=[0 0 0]  RotationSequenceAnglesUnits=deg  RotationMatrix=[1 0 0; 0 1 0; 0 0 1]
  BaseSolid : sm_lib/Body Elements/File Solid  ExtGeomFileName=01_BaseGP.STEP  UnitType=FromFile  ExtGeomFileUnits=m  StepReaderType=OCC  ExportConvexHullGeometry=off  InertiaType=Custom  Mass=307.29601379  MassUnits=kg  CenterOfMass=[0 -0.01488967 0.02139206]  CenterOfMassUnits=m  MomentsOfInertia=[29.78955950 5.25917100 29.30269608]  MomentsOfInertiaUnits=kg*m^2  ProductsOfInertia=[-3.89461427 -0.00003008 -0.00000910]  ProductsOfInertiaUnits=kg*m^2  BasedOnType=Density  Density=7300  DensityUnits=kg/m^3  DoExposeReferenceFrame=on  SerializedFrames=<Frames><Frame><Id>Frame1</Id><Value><Name>F2</Name><Origin><Source>GeometricFeature</Source><FeatureName>cylindrical surface 2</FeatureName></Origin><PrimaryAxis><DefinedDirection>+X</DefinedDirection><Source>ReferenceFrame</Source><SourceDirection>-Z</SourceDirection><FeatureName></FeatureName></PrimaryAxis><SecondaryAxis><DefinedDirection>+Y</DefinedDirection><Source>ReferenceFrame</Source><SourceDirection>+Y</SourceDirection><FeatureName></FeatureName></SecondaryAxis></Value></Frame><Frame><Id>Frame2</Id><Value><Name>F1</Name><Origin><Source>GeometricFeature</Source><FeatureName>cylindrical surface 1</FeatureName></Origin><PrimaryAxis><DefinedDirection>-X</DefinedDirection><Source>ReferenceFrame</Source><SourceDirection>+Z</SourceDirection><FeatureName></FeatureName></PrimaryAxis><SecondaryAxis><DefinedDirection>+Y</DefinedDirection><Source>ReferenceFrame</Source><SourceDirection>+Y</SourceDirection><FeatureName></FeatureName></SecondaryAxis></Value></Frame><Frame><Id>Frame3</Id><Value><Name>Bc1</Name><Origin><Source>GeometricFeature</Source><FeatureName>cylindrical surface 1</FeatureName></Origin><PrimaryAxis><DefinedDirection>+X</DefinedDirection><Source>GeometricFeature</Source><SourceDirection>+Z</SourceDirection><FeatureName>segment 135</FeatureName></PrimaryAxis><SecondaryAxis><DefinedDirection>+Y</DefinedDirection><Source>ReferenceFrame</Source><SourceDirection>+Z</SourceDirection><FeatureName></FeatureName></SecondaryAxis></Value></Frame></Frames>  GraphicType=FromGeometry  MarkerShape=Sphere  MarkerSize=10  GraphicVisPropType=SimpleVisualProperties  GraphicDiffuseColor=[134 134 71]/255  GraphicSpecularColor=[0.5 0.5 0.5 1.0]  GraphicAmbientColor=[0.15 0.15 0.15 1.0]  GraphicEmissiveColor=[0.0 0.0 0.0 1.0]  GraphicShininess=75  GraphicOpacity=1.0
  Sim-PS1 : nesl_utility/Simulink-PS Converter  PhysicalDomain=network_engine_domain  SubClassName=ps_input  LeftPortType=input  RightPortType=output  PseudoPeriodic=off  Frequencies=[]  NoiseDistribution=none  NoiseParameters=[]  Unit=rad  AffineConversion=off  FilteringAndDerivatives=provide  SimscapeFilterOrder=2  InputFilterTimeConstant=0.001  UdotUserProvided=2
  Sine Wave : Sin  Amplitude=Th1A*Th1f  Frequency=Th1f  Phase=pi/2  SampleTime=0
  Sine Wave1 : Sin  Amplitude=Th1A*Th1f*Th1f  Frequency=Th1f  Phase=pi  SampleTime=0
  Theta1-rotation : sm_lib/Joints/Revolute Joint  JointMode=Normal  SenseConstraintForce=off  SenseConstraintForceX=off  SenseConstraintForceY=off  SenseConstraintForceZ=off  SenseConstraintTorque=off  SenseConstraintTorqueX=off  SenseConstraintTorqueY=off  SenseConstraintTorqueZ=off  SenseTotalForce=off  SenseTotalForceX=off  SenseTotalForceY=off  SenseTotalForceZ=off  SenseTotalTorque=off  SenseTotalTorqueX=off  SenseTotalTorqueY=off  SenseTotalTorqueZ=off  CompositeWrenchDir=FollowerOnBase  CompositeWrenchFrame=BaseFrame  EquilibriumPosition=0  EquilibriumPositionUnits=deg  SpringStiffness=0  SpringStiffnessUnits=N*m/deg  DampingCoefficient=0  DampingCoefficientUnits=N*m/(deg/s)  TorqueActuationMode=NoTorque  MotionActuationMode=InputMotion  SensePosition=off  SenseVelocity=off  SenseAcceleration=off  SenseTorqueForce=off  SenseLowerLimitTorqueForce=off  SenseUpperLimitTorqueForce=off  LowerLimitSpecify=off  LowerLimitBound=-90  LowerLimitBoundUnits=deg  LowerLimitStiffness=1e4  LowerLimitStiffnessUnits=N*m/deg  LowerLimitDamping=10  LowerLimitDampingUnits=N*m/(deg/s)  LowerLimitTransitionRegionWidth=0.1  LowerLimitTransitionRegionWidthUnits=deg  UpperLimitSpecify=off  UpperLimitBound=90  UpperLimitBoundUnits=deg  UpperLimitStiffness=1e4  UpperLimitStiffnessUnits=N*m/deg  UpperLimitDamping=10  UpperLimitDampingUnits=N*m/(deg/s)  UpperLimitTransitionRegionWidth=0.1  UpperLimitTransitionRegionWidthUnits=deg  PositionTargetSpecify=on  PositionTargetPriority=High  PositionTargetValue=0  PositionTargetValueUnits=deg  VelocityTargetSpecify=off  VelocityTargetPriority=High  VelocityTargetValue=0  VelocityTargetValueUnits=deg/s
  W : PMIOPort  Side=Left
  F1 : PMIOPort  Port=2  Side=Right
  F2_rot : PMIOPort  Port=3  Side=Right
  Bc1 : PMIOPort  Port=4  Side=Right
  wires:
  Sine Wave/1 -> Sim-PS1/2
  Sine Wave1/1 -> Sim-PS1/3
  Theta1[rad]/1 -> Sim-PS1/1  "Theta1"
  connections:
  BaseR_To_W/LConn1 -- BaseSolid/RConn1
  W/RConn1 -- BaseR_To_W/RConn1
  Theta1-rotation/LConn1 -- BaseSolid/LConn1
  Sim-PS1/RConn1 -- Theta1-rotation/LConn2
  F2_rot/RConn1 -- Theta1-rotation/RConn1
  F1/RConn1 -- BaseSolid/LConn2
  Bc1/RConn1 -- BaseSolid/RConn2

== system SimForcesGP2017a/Hydraulic manipulator, Simscape/Bc1_V_SS ==
  Mux3 : Mux  Inputs=6
  PS-Simulink Converter{1..3,7..9} (6 alike) : nesl_utility/PS-Simulink Converter  PhysicalDomain=network_engine_domain  SubClassName=ps_output  LeftPortType=input  RightPortType=output  PseudoPeriodic=off  Frequencies=[]  Unit=inherit  AffineConversion=off
  Selector : Selector  InputPortWidth=6  IndexOptions=Index vector (dialog)  Indices=[4 5 6 1 2 3]  OutputSizes=1
  Transform Sensor3 : sm_lib/Frames and Transforms/Transform Sensor  MeasurementFrame=NonRotatingFollower  SenseAngle=off  SenseAxis=off  SenseAngle1=off  SenseAngle2=off  SenseAngle3=off  SenseQ=off  SenseR=off  SenseOmegaX=on  SenseOmegaY=on  SenseOmegaZ=on  SenseOmega1=off  SenseOmega2=off  SenseOmega3=off  SenseQDot=off  SenseRDot=off  SenseAlphaX=off  SenseAlphaY=off  SenseAlphaZ=off  SenseAlpha1=off  SenseAlpha2=off  SenseAlpha3=off  SenseQDDot=off  SenseRDDot=off  SenseX=off  SenseY=off  SenseZ=off  SenseRad=off  SenseAzim=off  SenseDist=off  SenseInc=off  SenseXDot=on  SenseYDot=on  SenseZDot=on  SenseRadDot=off  SenseAzimDot=off  SenseDistDot=off  SenseIncDot=off  SenseXDDot=off  SenseYDDot=off  SenseZDDot=off  SenseRadDDot=off  SenseAzimDDot=off  SenseDistDDot=off  SenseIncDDot=off
  Pillar_Bc1 : PMIOPort  Side=Right
  W : PMIOPort  Port=2  Side=Left
  Bc1_V_SS : Outport
  wires:
  PS-Simulink Converter1/1 -> Mux3/4
  PS-Simulink Converter8/1 -> Mux3/3
  PS-Simulink Converter9/1 -> Mux3/1
  PS-Simulink Converter2/1 -> Mux3/5
  PS-Simulink Converter3/1 -> Mux3/6
  PS-Simulink Converter7/1 -> Mux3/2
  Mux3/1 -> Selector/1
  Selector/1 -> Bc1_V_SS/1
  connections:
  Transform Sensor3/RConn1 -- Pillar_Bc1/RConn1
  Transform Sensor3/RConn6 -- PS-Simulink Converter2/LConn1
  PS-Simulink Converter9/LConn1 -- Transform Sensor3/RConn2
  PS-Simulink Converter7/LConn1 -- Transform Sensor3/RConn3
  Transform Sensor3/RConn4 -- PS-Simulink Converter8/LConn1
  Transform Sensor3/LConn1 -- W/RConn1
  PS-Simulink Converter3/LConn1 -- Transform Sensor3/RConn7
  Transform Sensor3/RConn5 -- PS-Simulink Converter1/LConn1

== system SimForcesGP2017a/Hydraulic manipulator, Simscape/Bc2_V_SS ==
  Mux3 : Mux  Inputs=6
  PS-Simulink Converter{1..3,7..9} (6 alike) : nesl_utility/PS-Simulink Converter  PhysicalDomain=network_engine_domain  SubClassName=ps_output  LeftPortType=input  RightPortType=output  PseudoPeriodic=off  Frequencies=[]  Unit=inherit  AffineConversion=off
  Selector1 : Selector  InputPortWidth=6  IndexOptions=Index vector (dialog)  Indices=[4 5 6 1 2 3]  OutputSizes=1
  Transform Sensor1 : sm_lib/Frames and Transforms/Transform Sensor  MeasurementFrame=NonRotatingFollower  SenseAngle=off  SenseAxis=off  SenseAngle1=off  SenseAngle2=off  SenseAngle3=off  SenseQ=off  SenseR=off  SenseOmegaX=on  SenseOmegaY=on  SenseOmegaZ=on  SenseOmega1=off  SenseOmega2=off  SenseOmega3=off  SenseQDot=off  SenseRDot=off  SenseAlphaX=off  SenseAlphaY=off  SenseAlphaZ=off  SenseAlpha1=off  SenseAlpha2=off  SenseAlpha3=off  SenseQDDot=off  SenseRDDot=off  SenseX=off  SenseY=off  SenseZ=off  SenseRad=off  SenseAzim=off  SenseDist=off  SenseInc=off  SenseXDot=on  SenseYDot=on  SenseZDot=on  SenseRadDot=off  SenseAzimDot=off  SenseDistDot=off  SenseIncDot=off  SenseXDDot=off  SenseYDDot=off  SenseZDDot=off  SenseRadDDot=off  SenseAzimDDot=off  SenseDistDDot=off  SenseIncDDot=off
  Lift_Bc2 : PMIOPort  Side=Right
  W : PMIOPort  Port=2  Side=Left
  Bc2_V_SS : Outport
  wires:
  Mux3/1 -> Selector1/1
  PS-Simulink Converter7/1 -> Mux3/2
  PS-Simulink Converter3/1 -> Mux3/6
  PS-Simulink Converter2/1 -> Mux3/5
  PS-Simulink Converter9/1 -> Mux3/1
  PS-Simulink Converter8/1 -> Mux3/3
  PS-Simulink Converter1/1 -> Mux3/4
  Selector1/1 -> Bc2_V_SS/1
  connections:
  Transform Sensor1/RConn5 -- PS-Simulink Converter1/LConn1
  Transform Sensor1/RConn7 -- PS-Simulink Converter3/LConn1
  Transform Sensor1/LConn1 -- W/RConn1
  Transform Sensor1/RConn4 -- PS-Simulink Converter8/LConn1
  Transform Sensor1/RConn3 -- PS-Simulink Converter7/LConn1
  Transform Sensor1/RConn2 -- PS-Simulink Converter9/LConn1
  Transform Sensor1/RConn6 -- PS-Simulink Converter2/LConn1
  Transform Sensor1/RConn1 -- Lift_Bc2/RConn1

== system SimForcesGP2017a/Hydraulic manipulator, Simscape/D22_V_SS ==
  Mux3 : Mux  Inputs=6
  PS-Simulink Converter{1..3,7..9} (6 alike) : nesl_utility/PS-Simulink Converter  PhysicalDomain=network_engine_domain  SubClassName=ps_output  LeftPortType=input  RightPortType=output  PseudoPeriodic=off  Frequencies=[]  Unit=inherit  AffineConversion=off
  Selector1 : Selector  InputPortWidth=6  IndexOptions=Index vector (dialog)  Indices=[4 5 6 1 2 3]  OutputSizes=1
  Transform Sensor1 : sm_lib/Frames and Transforms/Transform Sensor  MeasurementFrame=NonRotatingFollower  SenseAngle=off  SenseAxis=off  SenseAngle1=off  SenseAngle2=off  SenseAngle3=off  SenseQ=off  SenseR=off  SenseOmegaX=on  SenseOmegaY=on  SenseOmegaZ=on  SenseOmega1=off  SenseOmega2=off  SenseOmega3=off  SenseQDot=off  SenseRDot=off  SenseAlphaX=off  SenseAlphaY=off  SenseAlphaZ=off  SenseAlpha1=off  SenseAlpha2=off  SenseAlpha3=off  SenseQDDot=off  SenseRDDot=off  SenseX=off  SenseY=off  SenseZ=off  SenseRad=off  SenseAzim=off  SenseDist=off  SenseInc=off  SenseXDot=on  SenseYDot=on  SenseZDot=on  SenseRadDot=off  SenseAzimDot=off  SenseDistDot=off  SenseIncDot=off  SenseXDDot=off  SenseYDDot=off  SenseZDDot=off  SenseRadDDot=off  SenseAzimDDot=off  SenseDistDDot=off  SenseIncDDot=off
  Obj_D22 : PMIOPort  Side=Right
  W : PMIOPort  Port=2  Side=Left
  D22_V_SS : Outport
  wires:
  Selector1/1 -> D22_V_SS/1
  Mux3/1 -> Selector1/1
  PS-Simulink Converter7/1 -> Mux3/2
  PS-Simulink Converter3/1 -> Mux3/6
  PS-Simulink Converter2/1 -> Mux3/5
  PS-Simulink Converter9/1 -> Mux3/1
  PS-Simulink Converter8/1 -> Mux3/3
  PS-Simulink Converter1/1 -> Mux3/4
  connections:
  Transform Sensor1/RConn5 -- PS-Simulink Converter1/LConn1
  Transform Sensor1/RConn7 -- PS-Simulink Converter3/LConn1
  Transform Sensor1/LConn1 -- W/RConn1
  Transform Sensor1/RConn4 -- PS-Simulink Converter8/LConn1
  Transform Sensor1/RConn3 -- PS-Simulink Converter7/LConn1
  Transform Sensor1/RConn2 -- PS-Simulink Converter9/LConn1
  Transform Sensor1/RConn6 -- PS-Simulink Converter2/LConn1
  Transform Sensor1/RConn1 -- Obj_D22/RConn1

== system SimForcesGP2017a/Hydraulic manipulator, Simscape/EndMassObject ==
  EndObjectMass : sm_lib/Body Elements/File Solid  ExtGeomFileName=10_ObjectGP.STEP  UnitType=FromFile  ExtGeomFileUnits=m  StepReaderType=OCC  ExportConvexHullGeometry=off  InertiaType=Custom  Mass=570.18877059  MassUnits=kg  CenterOfMass=[2.16142487 0.01347152 0.06601658]  CenterOfMassUnits=m  MomentsOfInertia=[46.81220713 72.19317437 67.11012925]  MomentsOfInertiaUnits=kg*m^2  ProductsOfInertia=[0.04641137 0.08825278 0.37588204]  ProductsOfInertiaUnits=kg*m^2  BasedOnType=Density  Density=7850  DensityUnits=kg/m^3  DoExposeReferenceFrame=off  SerializedFrames=<Frames><Frame><Id>Frame1</Id><Value><Name>P32p</Name><Origin><Source>GeometricFeature</Source><FeatureName>circular curve 7</FeatureName></Origin><PrimaryAxis><DefinedDirection>+Y</DefinedDirection><Source>GeometricFeature</Source><SourceDirection>+Z</SourceDirection><FeatureName>segment 159</FeatureName></PrimaryAxis><SecondaryAxis><DefinedDirection>+X</DefinedDirection><Source>ReferenceFrame</Source><SourceDirection>+X</SourceDirection><FeatureName></FeatureName></SecondaryAxis></Value></Frame><Frame><Id>Frame2</Id><Value><Name>D22</Name><Origin><Source>GeometricFeature</Source><FeatureName>planar surface 154</FeatureName></Origin><PrimaryAxis><DefinedDirection>+Z</DefinedDirection><Source>ReferenceFrame</Source><SourceDirection>+Z</SourceDirection><FeatureName></FeatureName></PrimaryAxis><SecondaryAxis><DefinedDirection>+X</DefinedDirection><Source>ReferenceFrame</Source><SourceDirection>+X</SourceDirection><FeatureName></FeatureName></SecondaryAxis></Value></Frame></Frames>  GraphicType=FromGeometry  MarkerShape=Sphere  MarkerSize=10  GraphicVisPropType=SimpleVisualProperties  GraphicDiffuseColor=[255 9 134]/255  GraphicSpecularColor=[0.5 0.5 0.5 1.0]  GraphicAmbientColor=[0.15 0.15 0.15 1.0]  GraphicEmissiveColor=[0.0 0.0 0.0 1.0]  GraphicShininess=75  GraphicOpacity=1.0
  P32p_to_P32 : sm_lib/Frames and Transforms/Rigid Transform  TranslationMethod=StandardAxis  TranslationStandardOffset=17  TranslationLengthUnit=mm  TranslationStandardAxis=+Z  TranslationCartesianOffset=[0 0 0]  TranslationROffset=0  TranslationROffsetUnits=m  TranslationZOffset=0  TranslationZOffsetUnits=m  TranslationThetaOffset=0  TranslationThetaOffsetUnits=deg  RotationMethod=None  RotationAngleUnits=deg  RotationStandardAxis=+Y  RotationAngle=-90  RotationArbitraryAxis=[0 0 1]  FollAlignAxisA=+X  BaseAlignAxisA=+Y  FollAlignAxisB=+Y  BaseAlignAxisB=+Z  RotationSequenceAxes=FollowerAxes  RotationSequence=XYX  RotationSequenceAngles=[0 0 0]  RotationSequenceAnglesUnits=deg  RotationMatrix=[1 0 0; 0 1 0; 0 0 1]
  P32 : PMIOPort  Side=Left
  D22 : PMIOPort  Port=2  Side=Left
  connections:
  EndObjectMass/LConn1 -- P32p_to_P32/LConn1
  P32p_to_P32/RConn1 -- P32/RConn1
  D22/RConn1 -- EndObjectMass/RConn1
